simulink model "article_implementation"  (R2020b)
settings: Solver=VariableStepAuto  StartTime=0.0  StopTime=30  RelTol=1e-3
values from neighbouring files (symbols this model uses):
  C = [1 0]    [KalmanFilter.m]    (also in main.m = [eye(3), zeros(3,3)])
  Q = stat.C.gyro.var(1) * [1 0; 0 1/10]    [KalmanFilter.m]    (also in main.m = [Q_w, zeros(3,3);zeros(3,3), Q_b])
  R = 1/5 * stat.C.gyro.var(1)    [KalmanFilter.m]    (also in main.m = eye(3)*0.005)
settings Model: Creator=renato  LastModifiedBy=renato

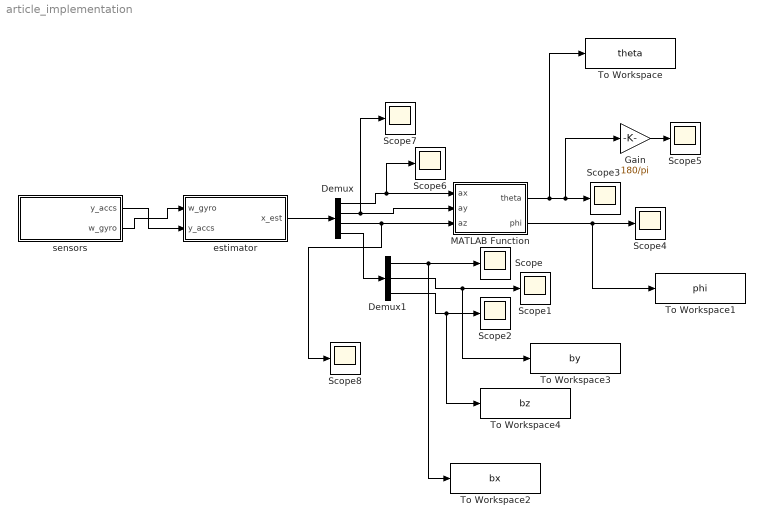
== system article_implementation ==
  Demux : Demux  Outputs=[1 1 1 3]
  Demux1 : Demux  Outputs=[1 1 1]
  Gain : Gain  Gain=180/pi
  MATLAB Function : MATLAB Function  TreatAsAtomicUnit=on
  Scope{,1..8} (9 alike) : Scope
  To Workspace : ToWorkspace  VariableName=theta  SaveFormat=Timeseries  SampleTime=-1
  To Workspace1 : ToWorkspace  VariableName=phi  SaveFormat=Timeseries  SampleTime=-1
  To Workspace2 : ToWorkspace  VariableName=bx  SaveFormat=Timeseries  SampleTime=-1
  To Workspace3 : ToWorkspace  VariableName=by  SaveFormat=Timeseries  SampleTime=-1
  To Workspace4 : ToWorkspace  VariableName=bz  SaveFormat=Timeseries  SampleTime=-1
  estimator : Subsystem
  sensors : Subsystem
  wires:
  estimator/1(x_est) -> Demux/1
  Demux/1 -> Scope6/1, MATLAB Function/1(ax)
  Demux/2 -> Scope7/1, MATLAB Function/2(ay)
  Demux/3 -> Scope8/1, MATLAB Function/3(az)
  Demux/4 -> Demux1/1
  Demux1/1 -> To Workspace2/1, Scope/1
  Demux1/3 -> To Workspace4/1, Scope2/1
  MATLAB Function/1(theta) -> To Workspace/1, Gain/1, Scope3/1
  MATLAB Function/2(phi) -> To Workspace1/1, Scope4/1
  sensors/1(y_accs) -> estimator/2(y_accs)
  sensors/2(w_gyro) -> estimator/1(w_gyro)
  Gain/1 -> Scope5/1
  Demux1/2 -> To Workspace3/1, Scope1/1

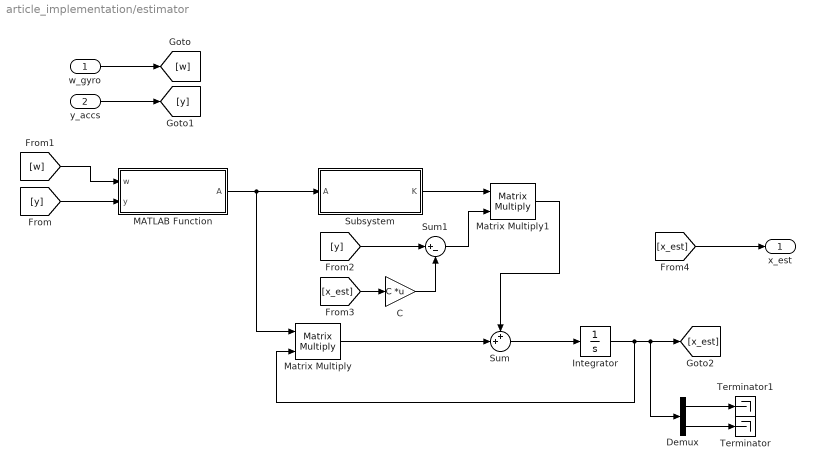
== system article_implementation/estimator ==
  w_gyro : Inport
  y_accs : Inport  Port=2
  C : Gain  Gain=C  Multiplication=Matrix(K*u)
  Demux : Demux  Outputs=[3 3]
  Integrator : Integrator
  MATLAB Function : MATLAB Function  TreatAsAtomicUnit=on
  Matrix Multiply : Product  Multiplication=Matrix(*)
  Matrix Multiply1 : Product  Multiplication=Matrix(*)
  Subsystem : Subsystem
  Sum : Sum  Inputs=++|
  Sum1 : Sum  Inputs=|+-
  Terminator : Terminator
  Terminator1 : Terminator
  x_est : Outport
  wires:
  Integrator/1 -> Demux/1, [x_est], Matrix Multiply/2
  Subsystem/1(K) -> Matrix Multiply1/1
  [x_est] -> C/1
  C/1 -> Sum1/2
  Sum/1 -> Integrator/1
  [y] -> MATLAB Function/2(y)
  [w] -> MATLAB Function/1(w)
  [y] -> Sum1/1
  Matrix Multiply1/1 -> Sum/1
  Sum1/1 -> Matrix Multiply1/2
  Matrix Multiply/1 -> Sum/2
  MATLAB Function/1(A) -> Subsystem/1(A), Matrix Multiply/1
  [x_est] -> x_est/1
  w_gyro/1 -> [w]
  y_accs/1 -> [y]
  Demux/2 -> Terminator/1
  Demux/1 -> Terminator1/1

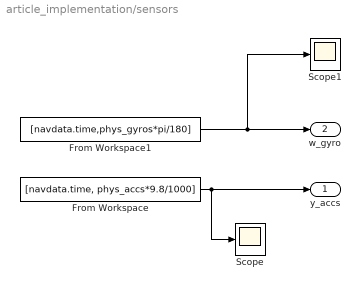
== system article_implementation/sensors ==
  From Workspace : FromWorkspace  VariableName=[navdata.time, phys_accs*9.8/1000]
  From Workspace1 : FromWorkspace  VariableName=[navdata.time,phys_gyros*pi/180]
  Scope : Scope
  Scope1 : Scope
  y_accs : Outport
  w_gyro : Outport  Port=2
  wires:
  From Workspace1/1 -> Scope1/1, w_gyro/1
  From Workspace/1 -> Scope/1, y_accs/1

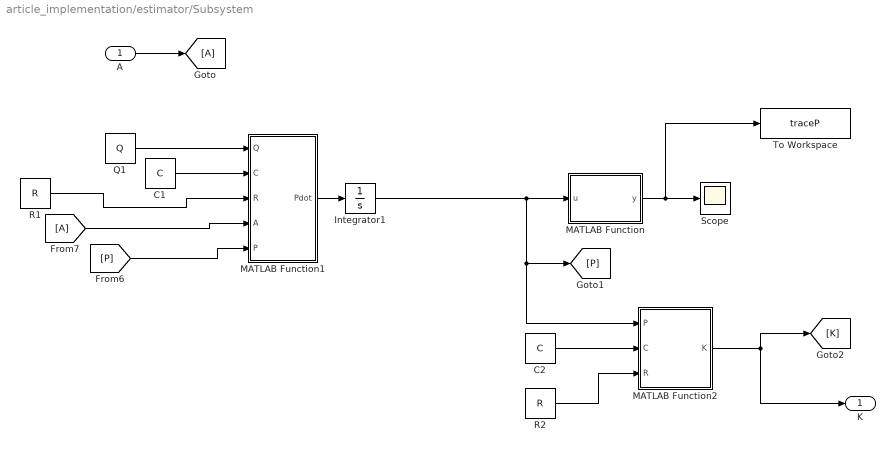
== system article_implementation/estimator/Subsystem ==
  A : Inport
  C1 : Constant  Value=C
  C2 : Constant  Value=C
  Integrator1 : Integrator  InitialCondition=eye(6)
  MATLAB Function : MATLAB Function  TreatAsAtomicUnit=on
  MATLAB Function1 : MATLAB Function  TreatAsAtomicUnit=on
  MATLAB Function2 : MATLAB Function  TreatAsAtomicUnit=on
  Q1 : Constant  Value=Q
  R1 : Constant  Value=R
  R2 : Constant  Value=R
  Scope : Scope
  To Workspace : ToWorkspace  VariableName=traceP  SaveFormat=Timeseries  SampleTime=-1
  K : Outport
  wires:
  A/1 -> [A]
  MATLAB Function/1(y) -> To Workspace/1, Scope/1
  Q1/1 -> MATLAB Function1/1(Q)
  [P] -> MATLAB Function1/5(P)
  [A] -> MATLAB Function1/4(A)
  R1/1 -> MATLAB Function1/3(R)
  C1/1 -> MATLAB Function1/2(C)
  MATLAB Function1/1(Pdot) -> Integrator1/1
  Integrator1/1 -> MATLAB Function2/1(P), [P], MATLAB Function/1(u)
  C2/1 -> MATLAB Function2/2(C)
  R2/1 -> MATLAB Function2/3(R)
  MATLAB Function2/1(K) -> [K], K/1

== matlab function article_implementation/MATLAB Function ==
  data: ax input; theta output; ay input; az input; phi output
function [theta, phi] = fcn(ax,ay,az)
    % need to see if the formulas are right
    %theta=atan2(ax, sqrt(az^2 + ay^2));
    theta=asin(ax/9.8);
    phi=atan(ay/az);

end

== matlab function article_implementation/estimator/MATLAB Function ==
  data: w input; A output; y input
function A = calculate_A(w, y)
    aux1 = -[0, -w(3), w(2); 
             w(3), 0, -w(1);
             -w(2), w(1), 0];
    aux2 = -[0, -y(3), y(2);
            y(3), 0, -y(1);
            -y(2), y(1), 0];   
    
A = [aux1 , aux2; zeros(3), zeros(3)];

== matlab function article_implementation/estimator/Subsystem/MATLAB Function ==
  data: u input; y output
function y = fcn(u)

y = trace(u);

== matlab function article_implementation/estimator/Subsystem/MATLAB Function1 ==
  data: Q input; Pdot output; C input; R input; A input; P input
function Pdot = fcn(Q,C,R,A,P)
    Pdot=A*P + P*A' +Q -P*C'/R*C*P;
end

== matlab function article_implementation/estimator/Subsystem/MATLAB Function2 ==
  data: P input; K output; C input; R input
function K = fcn(P,C,R)
    K=P*C'/R;
end
